simulink model "PIDTuningControl"  (R2017a)
settings: Solver=VariableStepAuto  StartTime=0.0  StopTime=duur  RelTol=1e-9  EnableMultiTasking=on
values from neighbouring files (symbols this model uses):
  K1 = 1    [PIDTuning.m]
  K2 = 3    [PIDTuning.m]    (also in margin.m)
  Kc = Kc_help(i)    [PIDTuning.m]    (also in PIDcontroller.m = 5; controlWithMeasurementDelay.m = 2)
  Km = 1    [PIDTuning.m]    (also in margin.m)
  tau1 = 2    [PIDTuning.m]    (also in PIDcontroller.m; margin.m)
  tau2 = 6    [PIDTuning.m]    (also in PIDcontroller.m; margin.m)
  taud = taud_help(i)    [PIDTuning.m]
  taui = taui_help(i)    [PIDTuning.m]
  taum = 0.2    [PIDTuning.m]    (also in margin.m)
libraries: simulink x1
settings Model: Creator=wrquaghe  LastModifiedBy=geert
settings DataIOCC: LimitDataPoints=on
settings OptimizationCC: LifeSpan=inf
settings DebuggingCC: AllowSymbolicDim=off  SFUnexpectedBacktrackingDiag=warning  SFNoUnconditionalDefaultTransitionDiag=warning  SFExecutionAtInitializationDiag=none
settings ModelReferenceCC: PropagateSignalLabelsOutOfModel=off
settings GRTTargetCC: TargetLangStandard=C89/C90 (ANSI)
settings ConfigComp: CovMetricSettings=dw  CovHtmlReporting=on  CovSaveCumulativeToWorkspaceVar=on  CovSaveSingleToWorkspaceVar=on  CovExternalEMLEnable=off

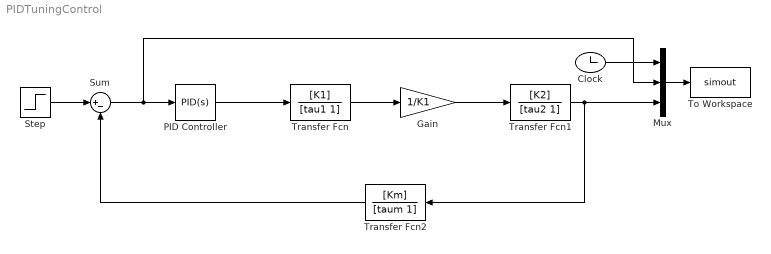
== system PIDTuningControl ==
  Clock : Clock
  Gain : Gain  Gain=1/K1
  Mux : Mux  Inputs=3
  PID Controller : simulink/Continuous/PID Controller  Controller=PID  TimeDomain=Continuous-time  SampleTime=-1  IntegratorMethod=Forward Euler  FilterMethod=Forward Euler  Form=Parallel  UseFilter=on  ControllerParametersSource=internal  P=Kc  I=Kc/taui  D=Kc*taud  N=100  InitialConditionSource=internal  InitialConditionForIntegrator=0  InitialConditionForFilter=0  ExternalReset=none  LimitOutput=off  UpperSaturationLimit=inf  LowerSaturationLimit=-inf  LinearizeAsGain=on  AntiWindupMode=none  Kb=1  TrackingMode=off  Kt=1  PParamMin=[]  PParamMax=[]  IParamMin=[]  IParamMax=[]  DParamMin=[]  DParamMax=[]  NParamMin=[]  NParamMax=[]  KbParamMin=[]  KbParamMax=[]  KtParamMin=[]  KtParamMax=[]  POutMin=[]  POutMax=[]  IOutMin=[]  IOutMax=[]  DOutMin=[]  DOutMax=[]  NOutMin=[]  NOutMax=[]  KbOutMin=[]  KbOutMax=[]  KtOutMin=[]  KtOutMax=[]  IntegratorOutMin=[]  IntegratorOutMax=[]  FilterOutMin=[]  FilterOutMax=[]  SumOutMin=[]  SumOutMax=[]  SumI1OutMin=[]  SumI1OutMax=[]  SumI2OutMin=[]  SumI2OutMax=[]  SumI3OutMin=[]  SumI3OutMax=[]  SumDOutMin=[]  SumDOutMax=[]  SaturationOutMin=[]  SaturationOutMax=[]  IntegratorContinuousStateAttributes=''  IntegratorStateMustResolveToSignalObject=off  IntegratorRTWStateStorageClass=Auto  FilterContinuousStateAttributes=''  FilterStateMustResolveToSignalObject=off  FilterRTWStateStorageClass=Auto  DifferentiatorICPrevScaledInput=0  DifferentiatorOutMin=[]  DifferentiatorOutMax=[]  InitialConditionSetting=State (most efficient)
  Step : Step  Time=0  SampleTime=0
  Sum : Sum  Inputs=|+-
  To Workspace : ToWorkspace  VariableName=simout  SampleTime=-1
  Transfer Fcn : TransferFcn  Numerator=[K1]  Denominator=[tau1 1]
  Transfer Fcn1 : TransferFcn  Numerator=[K2]  Denominator=[tau2 1]
  Transfer Fcn2 : TransferFcn  Numerator=[Km]  Denominator=[taum 1]
  wires:
  Sum/1 -> Mux/2, PID Controller/1
  Transfer Fcn/1 -> Gain/1
  Gain/1 -> Transfer Fcn1/1
  Transfer Fcn1/1 -> Transfer Fcn2/1, Mux/3
  Transfer Fcn2/1 -> Sum/2
  Clock/1 -> Mux/1
  Mux/1 -> To Workspace/1
  Step/1 -> Sum/1
  PID Controller/1 -> Transfer Fcn/1
